simulink model "FuelTimer_harness"  (Simulink 7.7)
settings: Solver=FixedStepDiscrete  SolverMode=SingleTasking  StartTime=0.0  StopTime=100  FixedStep=.01  RelTol=1e-3
PostLoadFcn:
  | cd '..';
  | PostLoadFcn;
  | cd 'harness';
InitFcn:
  | if signalbuilder('FuelTimer_harness/Signal Builder','activegroup') == 1
  |   CD_FUEL_PRIMARY_FUNCTION.DataType = 'uint8';
  |   CD_FUEL_PRIMARY_FUNCTION.Value = 255;
  | else
  |   CD_FUEL_PRIMARY_FUNCTION.DataType = 'uint8';
  |   CD_FUEL_PRIMARY_FUNCTION.Value = 0;
  | end
undefined symbols (not defined in the file): ACTIVE, CD_FUEL_RESOLUTION_TIMER, INACTIVE, NON_FUNCTIONAL, sigbuilder_block, srate100
settings Model: Creator=smindema  LastModifiedBy=aliebel  CovMetricSettings=dcmw  CovHTMLOptions=-aTS=1 -bRG=1 -bTC=1 -hTR=0 -nFC=0 -scm=1 -bcm=1 -xEv=0  covSaveCumulativeToWorkspaceVar=off  CovSaveSingleToWorkspaceVar=off
settings MATStruct: SampleTime=0.01  Offset=0  Priority=[1.0]
settings DataIOCC: LimitDataPoints=off  SaveOutput=off  SaveTime=off
settings OptimizationCC: BlockReduction=off  InlineParams=on  ExpressionFolding=off  StateBitsets=on  DataBitsets=on  UseTempVars=on  InitFltsAndDblsToZero=on  NoFixptDivByZeroProtection=on  EfficientFloat2IntCast=on  OptimizeModelRefInitCode=on
settings DebuggingCC: SaveWithParameterizedLinksMsg=none  MultiTaskDSMMsg=warning  MultiTaskCondExecSysMsg=none  IntegerOverflowMsg=none  ModelReferenceCSMismatchMessage=warning
settings HardwareCC: ProdBitPerInt=16  ProdBitPerPointer=16  ProdIntDivRoundTo=Floor  ProdEndianess=BigEndian  ProdWordSize=16  ProdHWDeviceType=Motorola HC12
settings ModelReferenceCC: ModelReferenceNumInstancesAllowed=Single
settings RTWCC: SystemTargetFile=ert.tlc  GenCodeOnly=on  TemplateMakefile=ert_default_tmf  Description=Real-Time Workshop Embedded Coder (no auto configuration)  GenerateReport=on  RetainRTWFile=on  ProcessScript=ert_make_rtw_hook  IncludeHyperlinkInReport=on  LaunchReport=on  IncludeERTFirstTime=on
settings RTWCC: CustomHeaderCode=|
  | #include "cpp_req_defines.h"
  | #include "hw_fin.h"
  | #include "cdata.h"
settings CodeAppCC: IgnoreCustomStorageClasses=off  DefineNamingRule=UpperCase
settings ERTTargetCC: TargetFcnLib=ansi_tfl_tmw.mat  FunctionExecutionProfile=off  MultiwordLength=2048  GenerateSampleERTMain=on  IncludeMdlTerminateFcn=off  SupportAbsoluteTime=off  SupportNonFinite=off  SupportComplex=off  PurelyIntegerCode=on  ERTCustomFileTemplate=gen_rtw_req_defines_h.tlc  GlobalDataDefinition=InSeparateSourceFile  GlobalDataReference=InSeparateHeaderFile  ConvertIfToSwitch=off

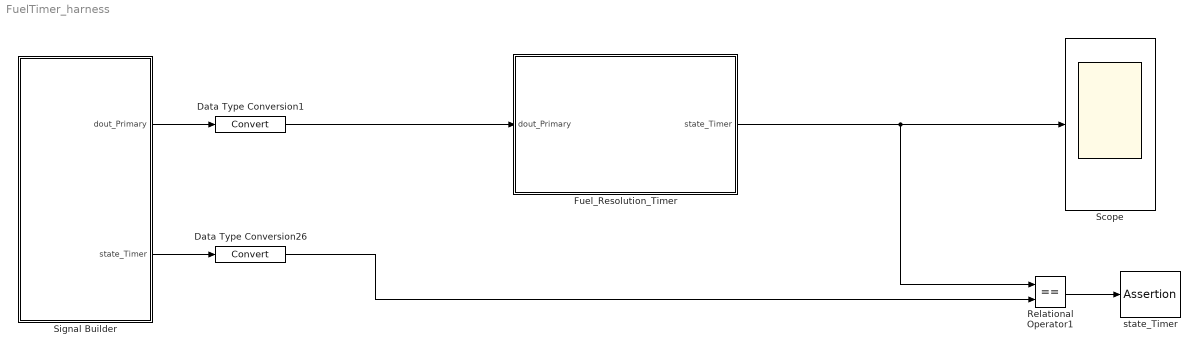
== system FuelTimer_harness ==
  Data Type Conversion1 : DataTypeConversion
  Data Type Conversion26 : DataTypeConversion
  Fuel_Resolution_Timer : Subsystem  TreatAsAtomicUnit=on  SystemSampleTime=srate100  RTWFileName=mod_Outputs  mask{CD_PRIMARY_FUNCTION=CD_FUEL_PRIMARY_FUNCTION, CD_RESOLUTION_TIMER=CD_FUEL_RESOLUTION_TIMER}
      mask prompts: CD_PRIMARY_FUNCTION "Primary Function"; CD_RESOLUTION_TIMER "Resolution Timer"
      settings: RTWSystemCode=Function  RTWFcnNameOpts=Use subsystem name  RTWFileNameOpts=User specified
  Relational Operator1 : RelationalOperator  Operator===  OutDataTypeStr=boolean
  Scope : Scope
      settings: TimeRange=100  YMin=0  YMax=6  DataFormat=Array
  Signal Builder : Subsystem  Tag=STV Subsys  LoadFcn=sigbuilder_block('load',[92.25 118.5 933.75 640.5 ]);  StartFcn=sigbuilder_block('start');  StopFcn=sigbuilder_block('stop');  ClipboardFcn=sigbuilder_block('clipboard');  mask(Sigbuilder block){}
      mask help: Create and generate interchangeable groups of signals whose waveforms are piecewise linear.
      mask init:
      | if ~strcmp(get_param(bdroot(gcbh),'SimulationStatus'),'stopped') tuvar = sigbuilder_block('maskInit'); end
      settings: CopyFcn=sigbuilder_block('copy');  DeleteFcn=sigbuilder_block('delete');  ModelCloseFcn=sigbuilder_block('modelClose');  PreSaveFcn=sigbuilder_block('preSave');  NameChangeFcn=sigbuilder_block('namechange');  OpenFcn=sigbuilder_block('open',[1440 133.5 1440 753 ]);  CloseFcn=sigbuilder_block('close');
      mask Display: plot(0, 0, 100, 100,[2, 2, 32, 32, 2], [68, 8, 8, 68, 68],[32, 2], [38, 38], [32, 19, 2],[53, 60, 44], [32, 17, 17, 2],[16, 16, 31, 31]);txt = getActiveGroup(gcbh);text(2, 100, txt,'verticalAlignment', 'top');
  state_Timer : Assertion  Enabled=on
  wires:
  Relational Operator1/1 -> state_Timer/1
  Data Type Conversion26/1 -> Relational Operator1/2
  Fuel_Resolution_Timer/1(state_Timer) -> Scope/1, Relational Operator1/1
  Signal Builder/1(dout_Primary) -> Data Type Conversion1/1
  Data Type Conversion1/1 -> Fuel_Resolution_Timer/1(dout_Primary)
  Signal Builder/2(state_Timer) -> Data Type Conversion26/1

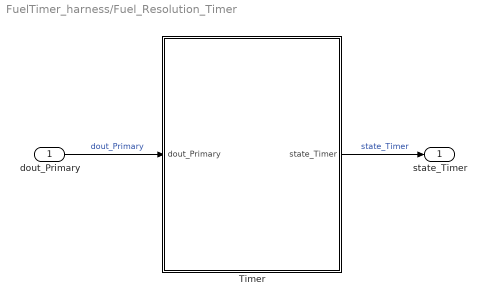
== system FuelTimer_harness/Fuel_Resolution_Timer ==
  dout_Primary : Inport
  Timer : Stateflow chart  TreatAsAtomicUnit=on
  state_Timer : Outport
  wires:
  Timer/1(state_Timer) -> state_Timer/1  "state_Timer"
  dout_Primary/1 -> Timer/1(dout_Primary)  "dout_Primary"

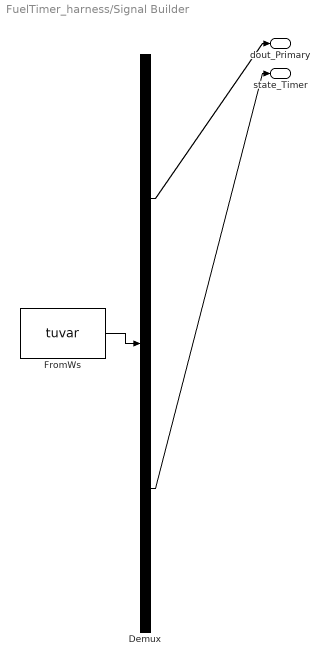
== system FuelTimer_harness/Signal Builder ==
  Demux : Demux  Tag=STV Demux  Outputs=2
  FromWs : FromWorkspace  Tag=STV FromWs  VariableName=tuvar  SampleTime=0  SigBuilderData=DataTag0  VnvData=DataTag1
      SigBuilderData=|
      | common.afterFinalStr = 'Extrapolate'
      | common.sampleTime = 0
      | dataSet(1).timeRange = [0 100]
      | dataSet(1).name = 'NonFunctional'
      | dataSet(2).timeRange = [0 100]
      | dataSet(2).name = 'Functional1'
      | sbobj.Groups(1).Name = 'NonFunctional'
      | sbobj.Groups(1).Signals(1).Name = 'dout_Primary'
      | sbobj.Groups(1).Signals(1).XData = [0 10.03 10.03 14.3 14.3 100]
      | sbobj.Groups(1).Signals(1).YData = [0 0 1 1 0 0]
      | sbobj.Groups(1).Signals(2).Name = 'state_Timer'
      | sbobj.Groups(1).Signals(2).XData = [0 32 39.2 100]
      | sbobj.Groups(1).Signals(2).YData = [0 0 0 0]
      | sbobj.Groups(1).TimeRange = [0 100]
      | sbobj.Groups(2).Name = 'Functional1'
      | sbobj.Groups(2).Signals(1).Name = 'dout_Primary'
      | sbobj.Groups(2).Signals(1).XData = [0 10.03 10.03 10.64 10.64 100]
      | sbobj.Groups(2).Signals(1).YData = [0 0 1 1 0 0]
      | sbobj.Groups(2).Signals(2).Name = 'state_Timer'
      | sbobj.Groups(2).Signals(2).XData = [0 10.7 10.7 15.8 15.8 100]
      | sbobj.Groups(2).Signals(2).YData = [0 0 1 1 0 0]
      | sbobj.Groups(2).TimeRange = [0 100]
  dout_Primary : Outport  Tag=STV Outport
  state_Timer : Outport  Tag=STV Outport  Port=2
  wires:
  FromWs/1 -> Demux/1
  Demux/1 -> dout_Primary/1
  Demux/2 -> state_Timer/1

== stateflow chart Fuel_Resolution_Timer/Timer ==
  state INACTIVE_WAIT
    en:resolutionTimer = CD_RESOLUTION_TIMER;
  state INACTIVE
    en:state_Timer = INACTIVE;
  state ACTIVE
    en:state_Timer = ACTIVE;
    du:resolutionTimer--;
  (default) -> INACTIVE
  INACTIVE -> INACTIVE_WAIT : [(CD_PRIMARY_FUNCTION != NON_FUNCTIONAL) && (dout_Primary != INACTIVE)]
  INACTIVE_WAIT -> ACTIVE : [dout_Primary == INACTIVE]
  ACTIVE -> INACTIVE : [(resolutionTimer <= 0)]
  data: dout_Primary input boolean; state_Timer output uint8; ACTIVE parameter uint8; INACTIVE parameter uint8; NON_FUNCTIONAL parameter uint8; CD_PRIMARY_FUNCTION parameter uint8; CD_RESOLUTION_TIMER parameter uint16; resolutionTimer local uint16
